simulink subsystem "controller_skeleton_FILTERED"  (R2023b)
settings: Solver=FixedStepDiscrete  StartTime=0.0  StopTime=10.0  RelTol=1e-3  EnableMultiTasking=on
undefined symbols (not defined in the file): tvs
settings Model: Creator=Inver  LastModifiedBy=Inver
settings SolverCC: AutoInsertRateTranBlk=on
settings DataIOCC: SaveOutput=off  SaveTime=off
settings OptimizationCC: DefaultParameterBehavior=Inlined  InlineInvariantSignals=on  EnhancedBackFolding=on  PassReuseOutputArgsAs=Individual arguments  StateBitsets=on  DataBitsets=on  ZeroExternalMemoryAtStartup=off  ZeroInternalMemoryAtStartup=off  NoFixptDivByZeroProtection=on  LifeSpan=1  OptimizeBlockOrder=speed  DifferentSizesBufferReuse=on  EfficientTunableParamExpr=on
settings DebuggingCC: ParameterTunabilityLossMsg=error
settings HardwareCC: ProdBitPerPointer=32  ProdBitPerSizeT=32  ProdBitPerPtrDiffT=32  ProdLargestAtomicFloat=None  ProdIntDivRoundTo=Floor  ProdWordSize=32  ProdHWDeviceType=Generic->Custom
settings SFSimCC: MATLABDynamicMemAlloc=off
settings RTWCC: Description=Embedded Coder  SystemTargetFile=ert.tlc  TLCOptions=-p0  GenCodeOnly=on  TemplateMakefile=ert_default_tmf  GenerateReport=on  RTWVerbose=off  IncludeHyperlinkInReport=on  LaunchReport=on
settings CodeAppCC: ForceParamTrailComments=on  IgnoreCustomStorageClasses=off  OperatorAnnotations=on  SimulinkDataObjDesc=on  SFDataObjDesc=on  CustomSymbolStrGlobalVar=rt$N$M  CustomSymbolStrType=$N$M  CustomSymbolStrFcn=$N$M$F  CustomSymbolStrMacro=$N$M  InsertBlockDesc=on
settings ERTTargetCC: TargetLangStandard=C99 (ISO)  CodeReplacementLibrary=ISO_C  GenerateSampleERTMain=on  IncludeMdlTerminateFcn=off  SuppressErrorStatus=on  SupportAbsoluteTime=off  PurelyIntegerCode=on  SupportNonFinite=off  SupportComplex=off  InlinedParameterPlacement=NonHierarchical  RootIOFormat=Structure reference  ERTCustomFileTemplate=example_file_process.tlc

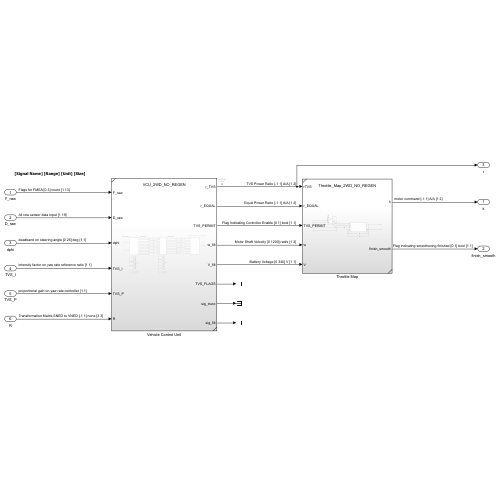
[thumbnail: Simulink's stored preview of the top-level diagram]
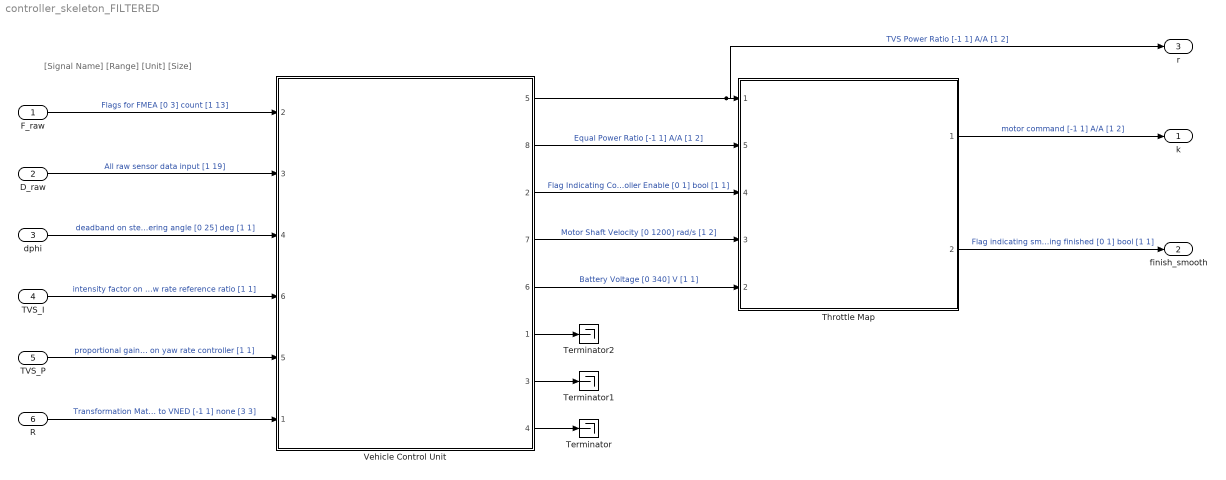
== system controller_skeleton_FILTERED ==
  note: [Signal Name] [Range] [Unit] [Size]
  F_raw : Inport
  D_raw : Inport  Port=2
  dphi : Inport  Port=3
  TVS_I : Inport  Port=4
  TVS_P : Inport  Port=5
  R : Inport  Port=6
  Terminator : Terminator
  Terminator1 : Terminator
  Terminator2 : Terminator
  Throttle Map : Subsystem  TreatAsAtomicUnit=on  SystemSampleTime=tvs.const.ts  ReferencedSubsystem=Throttle_Map_2WD_NO_REGEN
      settings: PortSchema="{\"entries\":[{\"content\":{\"sides\":[{\"content\":{\"connectorIds\":[\"In1\",\"In5\",\"In4\",\"In3\",\"In2\"]},\"type\":\"ConnectorPlacement.EquallySpacedRectSide\",\"uuid\":\"0a2325a3-9d51-4087-b02d-3e382446227a\"},{\"content\":{\"connectorIds\":[\"Out1\",\"Out2\"],\"side\":\"RIGHT\"},\"type\":\"ConnectorPlacement.EquallySpacedRectSide\",\"uuid\":\"1dae26bb-0e0b-4c8e-9d40-43caeaa44005\"},{\"content\":{\"side\":\"TOP\"},\"type\":\"ConnectorPlacement.EquallySpacedRectSide\",\"uuid\":\"12710057-5a58-45a8-acf5-4b6ffc7139ef\"}]},\"type\":\"ConnectorPlacement.EquallySpacedConnector\",\"uuid\":\"fad868a8-f7f5-4d78-95c0-434c459d05fc\"}],\"packageUris\":[\"http://schema.mathworks.com/mf0/Connector/R2020b\"],\"version\":\"1.0\"}"
  Vehicle Control Unit : Subsystem  TreatAsAtomicUnit=on  SystemSampleTime=tvs.const.ts  ReferencedSubsystem=VCU_2WD_NO_REGEN
      settings: PortSchema="{\"entries\":[{\"content\":{\"sides\":[{\"content\":{\"connectorIds\":[\"In2\",\"In3\",\"In4\",\"In6\",\"In5\",\"In1\"]},\"type\":\"ConnectorPlacement.EquallySpacedRectSide\",\"uuid\":\"0548fc7f-1908-4601-9b40-f103cb0729d1\"},{\"content\":{\"connectorIds\":[\"Out5\",\"Out8\",\"Out2\",\"Out7\",\"Out6\",\"Out1\",\"Out3\",\"Out4\"],\"side\":\"RIGHT\"},\"type\":\"ConnectorPlacement.EquallySpacedRectSide\",\"uuid\":\"44f548c0-6932-48d7-958b-e93fdf282eee\"},{\"content\":{\"side\":\"TOP\"},\"type\":\"ConnectorPlacement.EquallySpacedRectSide\",\"uuid\":\"cf24e617-7ee4-4f5a-ac95-d15b2dc6149d\"},{\"content\":{\"side\":\"BOTTOM\"},\"type\":\"ConnectorPlacement.EquallySpacedRectSide\",\"uuid\":\"873ea3c0-1709-4ff5-9735-309575c8ee2b\"}]},\"type\":\"ConnectorPlacement.EquallySpacedConnector\",\"uuid\":\"717fcefc-58f6-4eae-b182-8dc1a26bd962\"}],\"packageUris\":[\"http://schema.mathworks.com/mf0/Connector/R2020b\"],\"version\":\"1.0\"}"
  k : Outport
  finish_smooth : Outport  Port=2
  r : Outport  Port=3
  wires:
  Throttle Map/1 -> k/1  "motor command [-1 1] A/A [1 2]"
  Vehicle Control Unit/6 -> Throttle Map/2  "Battery Voltage [0 340] V [1 1]"
  Vehicle Control Unit/7 -> Throttle Map/3  "Motor Shaft Velocity [0 1200] rad/s [1 2]"
  R/1 -> Vehicle Control Unit/1  "Transformation Matrix SNED to VNED [-1 1] none [3 3]"
  Vehicle Control Unit/2 -> Throttle Map/4  "Flag Indicating Controller Enable [0 1] bool [1 1]"
  Vehicle Control Unit/5 -> Throttle Map/1, r/1  "TVS Power Ratio [-1 1] A/A [1 2]"
  F_raw/1 -> Vehicle Control Unit/2  "Flags for FMEA [0 3] count [1 13]"
  D_raw/1 -> Vehicle Control Unit/3  "All raw sensor data input [1 19]"
  TVS_I/1 -> Vehicle Control Unit/6  "intensity factor on yaw rate reference ratio [1 1]"
  dphi/1 -> Vehicle Control Unit/4  "deadband on steering angle [0 25] deg [1 1]"
  Vehicle Control Unit/8 -> Throttle Map/5  "Equal Power Ratio [-1 1] A/A [1 2]"
  Vehicle Control Unit/4 -> Terminator/1
  Vehicle Control Unit/3 -> Terminator1/1
  Vehicle Control Unit/1 -> Terminator2/1
  Throttle Map/2 -> finish_smooth/1  "Flag indicating smoothening finished [0 1] bool [1 1]"
  TVS_P/1 -> Vehicle Control Unit/5  "proportional gain on yaw rate controller [1 1]"
